simulink model "pendule_simple"  (R2016a)
settings: Solver=FixedStepAuto  StartTime=0.0  StopTime=1000  FixedStep=0.001  RelTol=1e-3
undefined symbols (not defined in the file): g, l
settings Model: Creator=nsurbayr  LastModifiedBy=nsurbayr

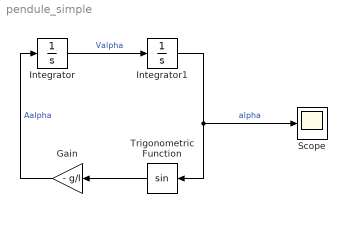
== system pendule_simple ==
  Gain : Gain  Gain=- g/l
  Integrator : Integrator
  Integrator1 : Integrator  InitialCondition=pi
  Scope : Scope
  Trigonometric Function : Trigonometry
  wires:
  Integrator/1 -> Integrator1/1  "Valpha"
  Gain/1 -> Integrator/1  "Aalpha"
  Trigonometric Function/1 -> Gain/1
  Integrator1/1 -> Scope/1, Trigonometric Function/1  "alpha"
